simulink model "scenario2"  (Simulink 9.1)
settings: Solver=VariableStepAuto  StartTime=0.0  StopTime=30  RelTol=1e-3
undefined symbols (not defined in the file or in its folder): sigbuilder_block
libraries: fuzblock x1
settings Model: Creator=Dimitris  LastModifiedBy=Dimitris
settings DataIOCC: SaveFormat=Dataset
settings OptimizationCC: LifeSpan=auto
settings DebuggingCC: UnderspecifiedInitializationDetection=Simplified  MergeDetectMultiDrivingBlocksExec=error  SFUnexpectedBacktrackingDiag=error  SFNoUnconditionalDefaultTransitionDiag=error  SFExecutionAtInitializationDiag=warning
settings HardwareCC: ProdBitPerPointer=64  ProdBitPerSizeT=64  ProdBitPerPtrDiffT=64  ProdLargestAtomicFloat=Float  ProdIntDivRoundTo=Zero  ProdEndianess=LittleEndian  ProdWordSize=64  ProdHWDeviceType=Intel->x86-64 (Windows64)
settings ModelReferenceCC: PropagateSignalLabelsOutOfModel=on
settings CodeAppCC: StateflowObjectComments=off
settings GRTTargetCC: TargetLangStandard=C99 (ISO)  CombineOutputUpdateFcns=on  GRTInterface=off
settings ConfigComp: CovMetricSettings=dwe  CovHtmlReporting=off  CovSaveCumulativeToWorkspaceVar=off  CovSaveSingleToWorkspaceVar=off  CovExternalEMLEnable=on

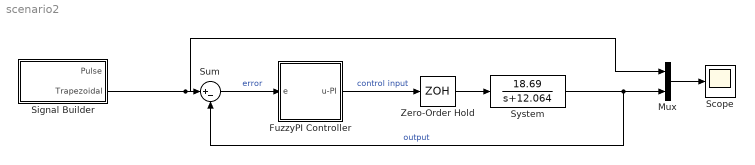
== system scenario2 ==
  FuzzyPI Controller : Subsystem
  Mux : Mux  Inputs=2
  Scope : Scope
  Signal Builder : Subsystem  Tag=STV Subsys  LoadFcn=sigbuilder_block('load');  StartFcn=sigbuilder_block('start');  StopFcn=sigbuilder_block('stop');  ClipboardFcn=sigbuilder_block('clipboard');  mask(Sigbuilder block){tuvar=[0:10]}
      mask help: Simulink:masks:SigbuilderBlock_MD
      mask init:
      | if ~strcmp(get_param(bdroot(gcbh),'SimulationStatus'),'stopped') tuvar = sigbuilder_block('maskInit'); end
      settings: CopyFcn=sigbuilder_block('copy');  DeleteFcn=sigbuilder_block('delete');  ModelCloseFcn=sigbuilder_block('modelClose');  PreSaveFcn=sigbuilder_block('preSave');  PauseFcn=sigbuilder_block('pause');  ContinueFcn=sigbuilder_block('continue');  NameChangeFcn=sigbuilder_block('namechange');  OpenFcn=sigbuilder_block('open',[60.75 181.5 633.75 477 ]);  CloseFcn=sigbuilder_block('close');
      mask Display: plot(0, 0, 100, 100,[2, 2, 32, 32, 2], [68, 8, 8, 68, 68],[32, 2], [38, 38], [32, 19, 2],[53, 60, 44], [32, 17, 17, 2],[16, 16, 31, 31]);txt = getActiveGroup(gcbh);text(2, 100, txt,'verticalAlignment', 'top');
  Sum : Sum  Inputs=|+-
  System : TransferFcn  Numerator=[18.69]  Denominator=[1 12.064]
  Zero-Order Hold : ZeroOrderHold  SampleTime=0.01
  wires:
  FuzzyPI Controller/1(u-PI) -> Zero-Order Hold/1  "control input"
  Mux/1 -> Scope/1
  Zero-Order Hold/1 -> System/1
  System/1 -> Mux/2, Sum/2  "output"
  Sum/1 -> FuzzyPI Controller/1(e)  "error"
  Signal Builder/2(Trapezoidal) -> Mux/1, Sum/1

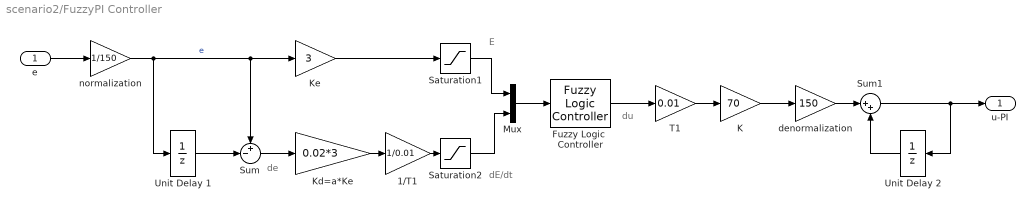
== system scenario2/FuzzyPI Controller ==
  note: E
  note: de
  note: dE/dt
  note: du
  e : Inport
  1/T1 : Gain  Gain=1/0.01
  "Fuzzy Logic  Controller " : fuzblock/Fuzzy Logic  Controller  FIS='FIS_COA.fis'  OutputSampleNumber=101  DataType=double  FuzzifiedInputs=off  RuleFiringStrengths=off  RuleOutputs=off  AggregatedOutputs=off  SimulateUsing=Interpreted execution  OutOfRangeInputValueMessage=warning  NoRuleFiredMessage=warning  EmptyOutputFuzzySetMessage=warning
  K : Gain  Gain=70
  Kd=a*Ke : Gain  Gain=0.02*3
  Ke : Gain  Gain=3
  Mux : Mux  Inputs=2
  Saturation1 : Saturate  UpperLimit=1  LowerLimit=-1
  Saturation2 : Saturate  UpperLimit=1  LowerLimit=-1
  Sum : Sum  Inputs=+-|
  Sum1 : Sum  Inputs=|++
  "T1 " : Gain  Gain=0.01
  Unit Delay 1 : UnitDelay  SampleTime=0.01
  Unit Delay 2 : UnitDelay  SampleTime=0.01
  denormalization : Gain  Gain=150
  normalization : Gain  Gain=1/150
  u-PI : Outport
  wires:
  e/1 -> normalization/1
  normalization/1 -> Unit Delay 1/1, Sum/1, Ke/1  "e"
  Unit Delay 1/1 -> Sum/2
  Sum/1 -> Kd=a*Ke/1
  Kd=a*Ke/1 -> 1/T1/1
  Ke/1 -> Saturation1/1
  1/T1/1 -> Saturation2/1
  Saturation1/1 -> Mux/1
  Saturation2/1 -> Mux/2
  "T1 "/1 -> K/1
  K/1 -> denormalization/1
  denormalization/1 -> Sum1/1
  Sum1/1 -> u-PI/1, Unit Delay 2/1
  Unit Delay 2/1 -> Sum1/2
  "Fuzzy Logic  Controller "/1 -> "T1 "/1
  Mux/1 -> "Fuzzy Logic  Controller "/1

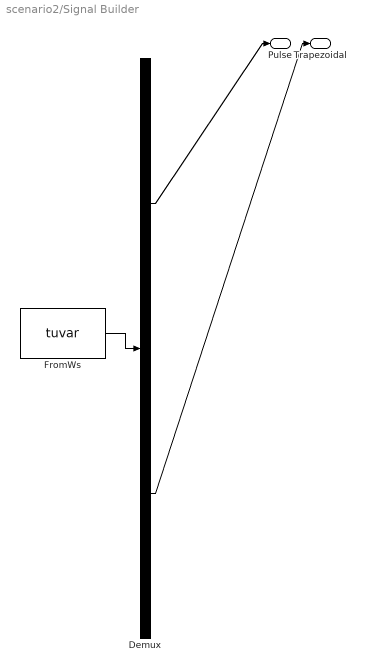
== system scenario2/Signal Builder ==
  Demux : Demux  Tag=STV Demux  Outputs=2
  FromWs : FromWorkspace  Tag=STV FromWs  VariableName=tuvar  SampleTime=0  SigBuilderData=DataTag0  VnvData=DataTag1
      SigBuilderData=|
      | common.afterFinalStr = 'Extrapolate'
      | common.sampleTime = 0
      | dataSet.timeRange = [0 30]
      | dataSet.name = 'Group 1'
      | sbobj.Groups.Name = 'Group 1'
      | sbobj.Groups.Signals(1).Name = 'Pulse'
      | sbobj.Groups.Signals(1).XData = [0 10.05 10.05 20 20 30]
      | sbobj.Groups.Signals(1).YData = [150 150 20 20 150 150]
      | sbobj.Groups.Signals(2).Name = 'Trapezoidal'
      | sbobj.Groups.Signals(2).XData = [0 10 20 30]
      | sbobj.Groups.Signals(2).YData = [0 150 150 0]
      | sbobj.Groups.TimeRange = [0 30]
  Pulse : Outport  Tag=STV Outport
  Trapezoidal : Outport  Tag=STV Outport  Port=2
  wires:
  FromWs/1 -> Demux/1
  Demux/1 -> Pulse/1
  Demux/2 -> Trapezoidal/1
